simulink model "pend"  (Simulink 4.00)
settings: Solver=ode45  StartTime=0.0  StopTime=60  RelTol=1e-3
settings Model: SaveState=on  SaveOutput=off  LimitDataPoints=off  ExtModeTrigMode=oneshot  ExtModeArmWhenConnect=off

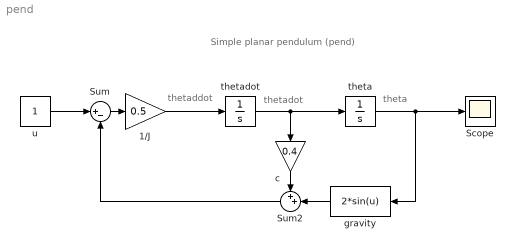
== system pend ==
  note: Simple planar pendulum (pend)
  note: thetadot
  note: theta
  note: thetaddot
  1/J : Gain  Gain=0.5  Multiplication=Element-wise(K.*u)  SaturateOnIntegerOverflow=on
  Scope : Scope
      settings: TimeRange=auto  YMin=-5  YMax=5  SaveToWorkspace=off  SaveName=ScopeData  LimitDataPoints=on  MaxDataPoints=5000
  Sum : Sum  Inputs=|+-  SaturateOnIntegerOverflow=on
  Sum2 : Sum  Orientation=left  Inputs=++|  SaturateOnIntegerOverflow=on
  c : Gain  Orientation=down  Gain=0.4  Multiplication=Element-wise(K.*u)  SaturateOnIntegerOverflow=on
  gravity : Fcn  Orientation=left  Expr=2*sin(u)
  theta : Integrator  ExternalReset=none  InitialConditionSource=internal  InitialCondition=0  LimitOutput=off  UpperSaturationLimit=inf  LowerSaturationLimit=-inf  ShowSaturationPort=off  ShowStatePort=off  AbsoluteTolerance=auto
  thetadot : Integrator  ExternalReset=none  InitialConditionSource=internal  InitialCondition=0  LimitOutput=off  UpperSaturationLimit=inf  LowerSaturationLimit=-inf  ShowSaturationPort=off  ShowStatePort=off  AbsoluteTolerance=auto
  u : Constant  Value=1
  wires:
  theta/1 -> gravity/1, Scope/1
  gravity/1 -> Sum2/2
  c/1 -> Sum2/1
  1/J/1 -> thetadot/1
  Sum/1 -> 1/J/1
  Sum2/1 -> Sum/2
  u/1 -> Sum/1
  thetadot/1 -> theta/1, c/1
